simulink model "modelB"  (R2019b)
settings: Solver=VariableStepAuto  StartTime=0.0  StopTime=10.0  RelTol=1e-3
libraries: fuzblock x1
settings Model: Creator=rafa  LastModifiedBy=rafa

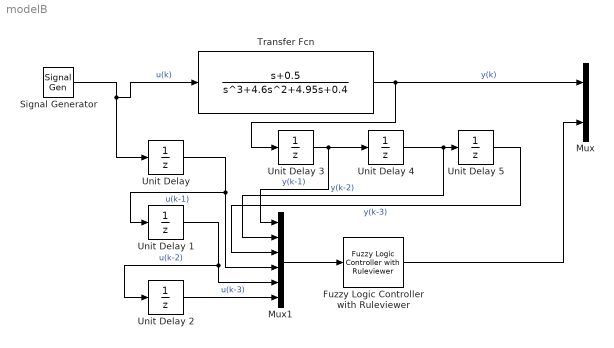
== system modelB ==
  "Fuzzy Logic Controller with Ruleviewer " : fuzblock/Fuzzy Logic  Controller  with Ruleviewer  fismatrix=myManualOptimizedFis.fis  Ts=24
  Mux : Mux  Inputs=2
  Mux1 : Mux  Inputs=6
  "Signal Generator " : SignalGenerator  Units=rad/sec
  Transfer Fcn : TransferFcn  Numerator=[1 0.5]  Denominator=[1 4.6 4.95 0.4]
  Unit Delay {,1..5} (6 alike) : UnitDelay  SampleTime=0.25  HasFrameUpgradeWarning=on
  wires:
  "Signal Generator "/1 -> "Unit Delay "/1, Transfer Fcn/1  "u(k)"
  "Unit Delay "/1 -> Mux1/4, Unit Delay 1/1  "u(k-1)"
  Unit Delay 1/1 -> Mux1/5, Unit Delay 2/1  "u(k-2)"
  Transfer Fcn/1 -> Unit Delay 3/1, Mux/1  "y(k)"
  Unit Delay 2/1 -> Mux1/6  "u(k-3)"
  Unit Delay 3/1 -> Unit Delay 4/1, Mux1/1  "y(k-1)"
  Unit Delay 4/1 -> Mux1/2, Unit Delay 5/1  "y(k-2)"
  "Fuzzy Logic Controller with Ruleviewer "/1 -> Mux/2
  Mux1/1 -> "Fuzzy Logic Controller with Ruleviewer "/1
  Unit Delay 5/1 -> Mux1/3  "y(k-3)"
